simulink model "mpc_demo"  (R2018b)
settings: Solver=ode45  StartTime=0.0  StopTime=20.0  MaxStep=0.01  RelTol=1e-3  EnableMultiTasking=on
libraries: simulink x1
settings Model: Creator=jgillis  LastModifiedBy=jgillis
settings DataIOCC: LimitDataPoints=on  SaveFormat=Array
settings OptimizationCC: LifeSpan=inf
settings DebuggingCC: SolverPrmCheckMsg=warning  SFUnexpectedBacktrackingDiag=warning  SFNoUnconditionalDefaultTransitionDiag=warning  SFExecutionAtInitializationDiag=none
settings HardwareCC: ProdBitPerPointer=32  ProdBitPerSizeT=32  ProdBitPerPtrDiffT=32  ProdLargestAtomicFloat=None  ProdIntDivRoundTo=Undefined  ProdEndianess=Unspecified  ProdWordSize=32  ProdHWDeviceType=32-bit Generic
settings ModelReferenceCC: PropagateSignalLabelsOutOfModel=off
settings SFSimCC: SimUseLocalCustomCode=off
settings RTWCC: RTWUseLocalCustomCode=off
settings CodeAppCC: StateflowObjectComments=on
settings GRTTargetCC: TargetLangStandard=C89/C90 (ANSI)  GeneratePreprocessorConditionals=Disable all
settings ConfigComp: CovMetricSettings=dw  CovHtmlReporting=on  CovSaveCumulativeToWorkspaceVar=on  CovSaveSingleToWorkspaceVar=on  CovExternalEMLEnable=off  CovSFcnEnable=off

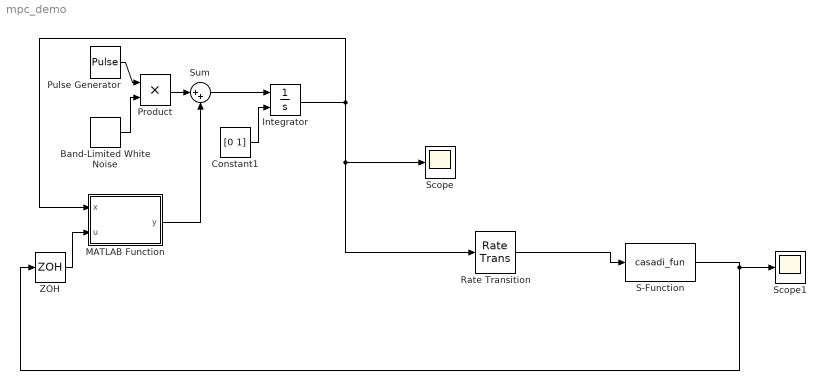
== system mpc_demo ==
  Band-Limited White Noise : simulink/Sources/Band-Limited White Noise  Cov=[1]  Ts=10  seed=[23341]
  Constant1 : Constant  Value=[0 1]
  Integrator : Integrator  InitialConditionSource=external  InitialCondition=[1 0]'
  MATLAB Function : MATLAB Function  TreatAsAtomicUnit=on
  Product : Product
  Pulse Generator : DiscretePulseGenerator  PulseType=Time based  Period=10  PulseWidth=5  PhaseDelay=10
  Rate Transition : RateTransition  OutPortSampleTime=0.5
  S-Function : S-Function  FunctionName=casadi_fun  Parameters='f.casadi', 'f'  SFunctionDeploymentMode=off  EnableBusSupport=off
  Scope : Scope
  Scope1 : Scope
  Sum : Sum  Inputs=|++
  ZOH : ZeroOrderHold  SampleTime=0.5
  wires:
  MATLAB Function/1(y) -> Sum/2
  Integrator/1 -> MATLAB Function/1(x), Rate Transition/1, Scope/1
  Constant1/1 -> Integrator/2
  S-Function/1 -> Scope1/1, ZOH/1
  ZOH/1 -> MATLAB Function/2(u)
  Rate Transition/1 -> S-Function/1
  Sum/1 -> Integrator/1
  Band-Limited White Noise/1 -> Product/2
  Product/1 -> Sum/1
  Pulse Generator/1 -> Product/1

== matlab function mpc_demo/MATLAB Function ==
  data: x input; u input; y output
function y = rhs(x,u)
%#codegen

y = [(1-x(2)^2)*x(1) - x(2) + u; x(1)];


end
